simulink model "completePathFollower"  (R2019a)
settings: Solver=ode4  StartTime=0.0  StopTime=100  FixedStep=P.Ts  RelTol=1e-3
undefined symbols (not defined in the file or in its folder): autopilot, desiredPath, forces_moments, P, true_states
libraries: simulink x3
settings Model: Creator=simao  LastModifiedBy=josea

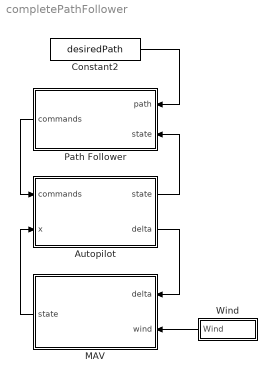
== system completePathFollower ==
  Autopilot : Subsystem
      mask Display: image(imread('../autopilot/simulink_imgs/kestrel.jpg'));
  Constant2 : Constant  Value=desiredPath
  MAV : Subsystem
      mask Display: image(imread('../autopilot/simulink_imgs/batcam.png'));
  Path Follower : Subsystem
      mask Display: image(imread('pathFollower_simulink_imgs/pathFollower_mask.png'));
  Wind : Subsystem
  wires:
  Constant2/1 -> Path Follower/1(path)
  Wind/1(Wind) -> MAV/2(wind)
  Autopilot/2(delta) -> MAV/1(delta)
  Autopilot/1(state) -> Path Follower/2(state)
  Path Follower/1(commands) -> Autopilot/1(commands)
  MAV/1(state) -> Autopilot/2(x)

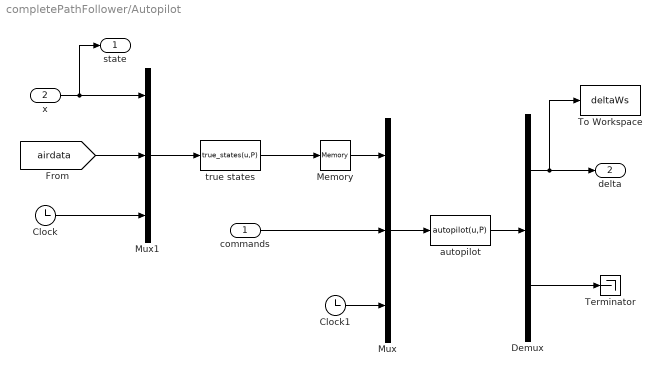
== system completePathFollower/Autopilot ==
  commands : Inport
  x : Inport  Port=2
  Clock : Clock
  Clock1 : Clock
  Demux : Demux  Outputs=[4;2]
  Memory : Memory
  Mux : Mux  Inputs=3
  Mux1 : Mux  Inputs=3
  Terminator : Terminator
  To Workspace : ToWorkspace  VariableName=deltaWs  SampleTime=-1
  autopilot : MATLABFcn  MATLABFcn=autopilot(u,P)  OutputDimensions=4+2  SampleTime=P.Ts
  true states : MATLABFcn  MATLABFcn=true_states(u,P)  OutputDimensions=19  SampleTime=P.Ts
  state : Outport
  delta : Outport  Port=2
  wires:
  Mux/1 -> autopilot/1
  Clock/1 -> Mux1/3
  autopilot/1 -> Demux/1
  Demux/1 -> To Workspace/1, delta/1
  Demux/2 -> Terminator/1
  commands/1 -> Mux/2
  Mux1/1 -> true states/1
  x/1 -> state/1, Mux1/1
  true states/1 -> Memory/1
  [airdata] -> Mux1/2
  Memory/1 -> Mux/1
  Clock1/1 -> Mux/3

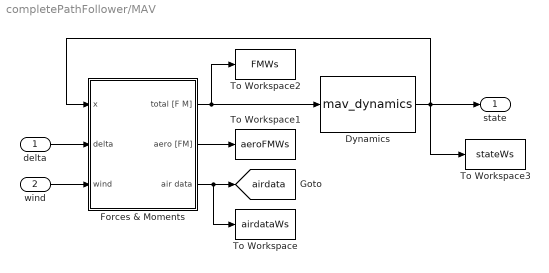
== system completePathFollower/MAV ==
  delta : Inport
  wind : Inport  Port=2
  Dynamics : S-Function  FunctionName=mav_dynamics  Parameters=P  SFunctionDeploymentMode=off  EnableBusSupport=off
  Forces & Moments : Subsystem
  To Workspace : ToWorkspace  VariableName=airdataWs  SampleTime=-1
  To Workspace1 : ToWorkspace  VariableName=aeroFMWs  SampleTime=-1
  To Workspace2 : ToWorkspace  VariableName=FMWs  SampleTime=-1
  To Workspace3 : ToWorkspace  VariableName=stateWs  SampleTime=-1
  state : Outport
  tag scope: airdata=global
  wires:
  Dynamics/1 -> To Workspace3/1, state/1, Forces & Moments/1(x)
  Forces & Moments/1(total [F M]) -> To Workspace2/1, Dynamics/1
  Forces & Moments/3(air data) -> [airdata], To Workspace/1
  delta/1 -> Forces & Moments/2(delta)
  wind/1 -> Forces & Moments/3(wind)
  Forces & Moments/2(aero [FM]) -> To Workspace1/1

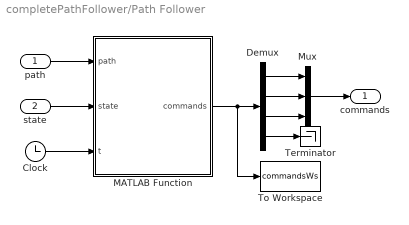
== system completePathFollower/Path Follower ==
  path : Inport
  state : Inport  Port=2
  Clock : Clock
  Demux : Demux
  MATLAB Function : MATLAB Function  TreatAsAtomicUnit=on
  Mux : Mux  Inputs=3
  Terminator : Terminator
  To Workspace : ToWorkspace  VariableName=commandsWs  SampleTime=-1
  commands : Outport
  wires:
  MATLAB Function/1(commands) -> Demux/1, To Workspace/1
  path/1 -> MATLAB Function/1(path)
  Clock/1 -> MATLAB Function/3(t)
  state/1 -> MATLAB Function/2(state)
  Demux/1 -> Mux/1
  Demux/2 -> Mux/2
  Demux/3 -> Mux/3
  Demux/4 -> Terminator/1
  Mux/1 -> commands/1

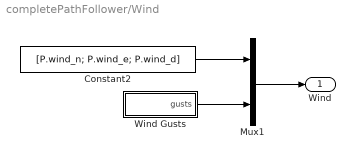
== system completePathFollower/Wind ==
  Constant2 : Constant  Value=[P.wind_n; P.wind_e; P.wind_d]
  Mux1 : Mux  Inputs=2
  Wind Gusts : Subsystem
  Wind : Outport
  wires:
  Constant2/1 -> Mux1/1
  Mux1/1 -> Wind/1
  Wind Gusts/1(gusts) -> Mux1/2

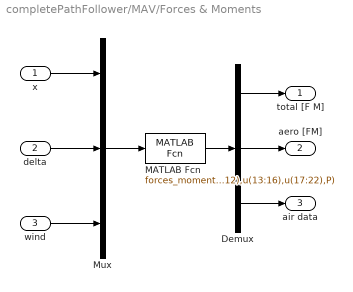
== system completePathFollower/MAV/Forces & Moments ==
  x : Inport
  delta : Inport  Port=2
  wind : Inport  Port=3
  Demux : Demux  Outputs=[6;6;6]
  MATLAB Fcn : MATLABFcn  MATLABFcn=forces_moments(u(1:12),u(13:16),u(17:22),P)  OutputDimensions=18
  Mux : Mux  Inputs=3
  total [F M] : Outport
  aero [FM] : Outport  Port=2
  air data : Outport  Port=3
  wires:
  Mux/1 -> MATLAB Fcn/1
  Demux/1 -> total [F M]/1
  MATLAB Fcn/1 -> Demux/1
  wind/1 -> Mux/3
  delta/1 -> Mux/2
  x/1 -> Mux/1
  Demux/3 -> air data/1
  Demux/2 -> aero [FM]/1

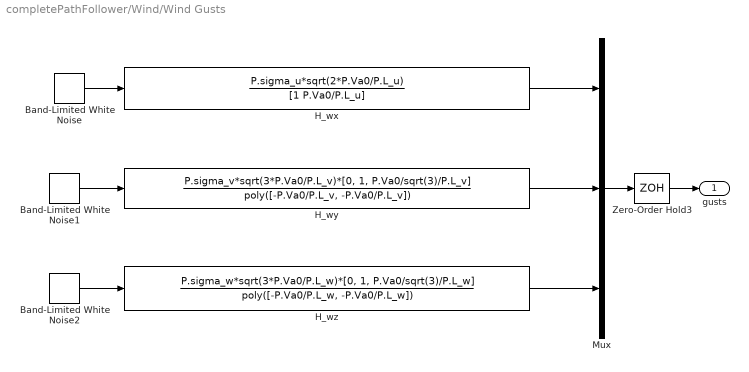
== system completePathFollower/Wind/Wind Gusts ==
  Band-Limited White Noise : simulink/Sources/Band-Limited White Noise  Cov=[1]  Ts=P.Ts  seed=[23341]
  Band-Limited White Noise1 : simulink/Sources/Band-Limited White Noise  Cov=[1]  Ts=P.Ts  seed=[23341]
  Band-Limited White Noise2 : simulink/Sources/Band-Limited White Noise  Cov=[1]  Ts=P.Ts  seed=[23341]
  H_wx : TransferFcn  Numerator=P.sigma_u*sqrt(2*P.Va0/P.L_u)  Denominator=[1 P.Va0/P.L_u]
  H_wy : TransferFcn  Numerator=P.sigma_v*sqrt(3*P.Va0/P.L_v)*[0, 1, P.Va0/sqrt(3)/P.L_v]  Denominator=poly([-P.Va0/P.L_v, -P.Va0/P.L_v])
  H_wz : TransferFcn  Numerator=P.sigma_w*sqrt(3*P.Va0/P.L_w)*[0, 1, P.Va0/sqrt(3)/P.L_w]  Denominator=poly([-P.Va0/P.L_w, -P.Va0/P.L_w])
  Mux : Mux  Inputs=3
  Zero-Order Hold3 : ZeroOrderHold  SampleTime=P.Ts
  gusts : Outport
  wires:
  H_wx/1 -> Mux/1
  Band-Limited White Noise/1 -> H_wx/1
  H_wy/1 -> Mux/2
  Band-Limited White Noise1/1 -> H_wy/1
  H_wz/1 -> Mux/3
  Band-Limited White Noise2/1 -> H_wz/1
  Mux/1 -> Zero-Order Hold3/1
  Zero-Order Hold3/1 -> gusts/1

== matlab function completePathFollower/Path Follower/MATLAB Function ==
  data: path input; state input; t input; commands output; P parameter
% path follow
%  - follow straight line path or orbit
%
% Modified:
%
% input is:
%   flag - if flag==1, follow waypoint path
%          if flag==2, follow orbit
%   
%   Va^d   - desired airspeed
%   r      - inertial position of start of waypoint path
%   q      - unit vector that defines inertial direction of waypoint path
%   c      - center of orbit
%   rho    - radius of orbit
%   lambda - direction of orbit (+1 for CW, -1 for CCW)
%   xhat   - estimated MAV states (pn, pe, pd, Va, alpha, beta, phi, theta, chi, p, q, r, Vg, wn, we, psi)
%
% output is:
%  Va_c - airspeed command
%  h_c  - altitude command
%  chi_c - heading command
%  phi_ff - feed forward roll command
%
function commands = path_follower(path,state,t,P)
    % path following gains
    chi_infty = 0.4;   % approach angle for large distance from straight-line path
    k_path    = 0.1;   % proportional gain for path following
    k_orbit   = 5;   % proportional gain for orbit following
%   gravity   = P.gravity;

    flag = path(1);   
    Va_d = path(2);
    
    rn = path(3);
    re = path(4);
    rd = path(5);
    
    qn = path(6);
    qe = path(7);
    qd = path(8);
    
    cn = path(9);
    ce = path(10);
    cd = path(11);
    
    rho_orbit = path(12);
    lam_orbit = path(13);
    
    pn     = state(1);
    pe     = state(2);
    pd     = state(3);
    psi    = state(9);
    
    chi = atan2(Va_d*sin(psi)+P.wind_e, Va_d*cos(psi)+P.wind_n);
    
    if flag == 1 % follow straight line path specified by r and q
        % compute wrapped version of path angle
        chi_q = atan2(qe,qn);
        while (chi_q - chi < -pi), chi_q = chi_q + 2*pi; end
        while (chi_q - chi > +pi), chi_q = chi_q - 2*pi; end

        e_py = -sin(chi_q)*(pn - rn) + cos(chi_q)*(pe - re);

        % heading command
        chi_c = chi_q - chi_infty*(2/pi)*atan(k_path*e_py);

        % commanded altitude

        e_p = [pn-rn; pe-re; pd-rd];

        n = [qe; -qn;0];
        n = n/norm(n);

        s = e_p - (dot(e_p,n))*n;

        sn = s(1);
        se = s(2);

        h_c = -rd - sqrt(sn^2 + se^2)*(qd/(sqrt(qn^2 + qe^2)));

        % roll feedforward command
        phi_ff = 0;
    else
        d = sqrt((pn - cn)^2 + (pe - ce)^2); % distance from orbit center, alterar

        % compute wrapped version of angular position on orbit
        varphi = atan2(pe - ce,pn - cn); %alterar
        while (varphi - chi < -pi), varphi = varphi + 2*pi; end
        while (varphi - chi > +pi), varphi = varphi - 2*pi; end

        % heading command      
        chi_c = varphi + lam_orbit*(pi/2+atan(k_orbit*(d-rho_orbit)/rho_orbit)) ; %alterar

        % commanded altitude is the height of the orbit
        h_c = -cd;

        % the roll angle feedforward command 
        phi_ff = 0;
    end
  
    % command airspeed equal to desired airspeed
    Va_c = Va_d;
  
    % create output
    commands = [Va_c; h_c; chi_c; phi_ff];
end
